simulink model "segway_planar_sim"  (R2023a)
settings: Solver=VariableStepAuto  StartTime=0.0  StopTime=5.0  RelTol=1e-3
values from neighbouring files (symbols this model uses):
  Cr2w = Cw2r^-1    [segway_ini.m]    (also in segway_planar_ini.m)
  Cw2r = [p.r/2     p.r/2;          p.r/p.b, -p.r/p.b]    [segway_ini.m]    (also in segway_planar_ini.m = [p.r])
  Ki = K(:,5:6)    [segway_ini.m]    (also in segway_planar_ini.m = K(:,4))
  Kx = K(:,1:4)    [segway_ini.m]    (also in segway_planar_ini.m = K(:,1:3))
  p = get_segway_params()    [segway_ini.m]    (also in segway_planar_ini.m)
  s = 2*pi    (= 6.28318530718)    [segway_planar_ini.m]
libraries: cstblocks x2
settings Model: Creator=Michael Peter  LastModifiedBy=Michael Peter

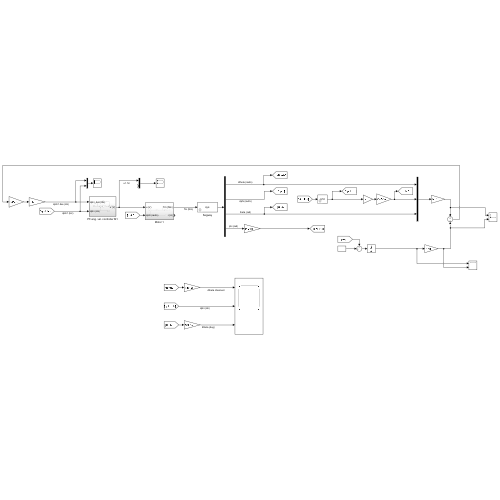
[thumbnail: Simulink's stored preview of the top-level diagram]
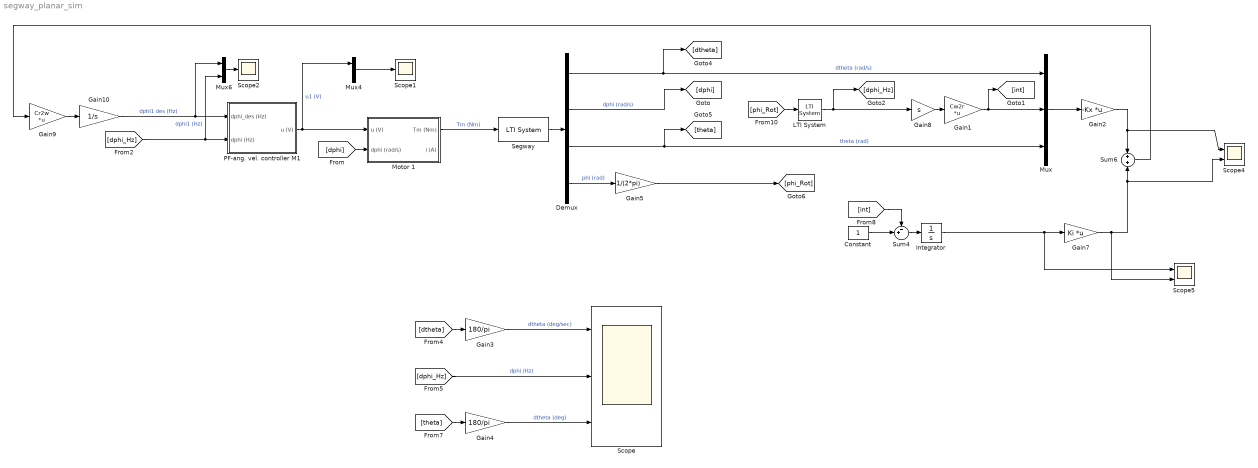
== system segway_planar_sim ==
  Constant : Constant
  Demux : Demux
  Gain1 : Gain  Gain=Cw2r  Multiplication=Matrix(K*u)
  Gain10 : Gain  Gain=1/s
  Gain2 : Gain  Gain=-Kx  Multiplication=Matrix(K*u)
  Gain3 : Gain  Gain=180/pi
  Gain4 : Gain  Gain=180/pi
  Gain5 : Gain  Gain=1/(2*pi)
  Gain7 : Gain  Gain=Ki  Multiplication=Matrix(K*u)
  Gain8 : Gain  Gain=s
  Gain9 : Gain  Gain=Cr2w  Multiplication=Matrix(K*u)
  Integrator : Integrator
  LTI System : cstblocks/LTI System  sys=Gfd  IC=[]
  Motor 1 : Subsystem
  Mux : Mux  Inputs=3
  Mux4 : Mux  Inputs=2
  Mux6 : Mux  Inputs=2
  PF-ang. vel. controller M1 : Subsystem
  Scope : Scope  NumInputPorts=3
  Scope1 : Scope
  Scope2 : Scope
  Scope4 : Scope  NumInputPorts=2
  Scope5 : Scope  NumInputPorts=2
  Segway : cstblocks/LTI System  sys=sys  IC=x0
  Sum4 : Sum  Inputs=-+|
  Sum6 : Sum  Inputs=+|+
  wires:
  Mux/1 -> Gain2/1
  Demux/2 -> [dphi]  "dphi (rad/s)"
  Segway/1 -> Demux/1
  Demux/3 -> [theta], Mux/3  "theta (rad)"
  Demux/1 -> [dtheta], Mux/1  "dtheta (rad/s)"
  Demux/4 -> Gain5/1  "phi (rad)"
  Sum4/1 -> Integrator/1
  Integrator/1 -> Scope5/1, Gain7/1
  [dtheta] -> Gain3/1
  [dphi_Hz] -> Scope/2  "dphi (Hz)"
  [theta] -> Gain4/1
  Gain3/1 -> Scope/1  "dtheta (deg/sec)"
  Gain4/1 -> Scope/3  "dtheta (deg)"
  Gain7/1 -> Scope5/2, Scope4/2, Sum6/2
  [int] -> Sum4/1
  [phi_Rot] -> LTI System/1
  Gain2/1 -> Sum6/1, Scope4/1
  LTI System/1 -> Gain8/1, [dphi_Hz]
  Constant/1 -> Sum4/2
  Sum6/1 -> Gain9/1
  Mux6/1 -> Scope2/1
  Motor 1/1(Tm (Nm)) -> Segway/1  "Tm (Nm)"
  PF-ang. vel. controller M1/1(u (V)) -> Mux4/1, Motor 1/1(u (V))  "u1 (V)"
  [dphi_Hz] -> PF-ang. vel. controller M1/2(dphi (Hz)), Mux6/2  "dphi1 (Hz)"
  Gain10/1 -> PF-ang. vel. controller M1/1(dphi_des (Hz)), Mux6/1  "dphi1 des (Hz)"
  [dphi] -> Motor 1/2(dphi (rad/s))
  Mux4/1 -> Scope1/1
  Gain8/1 -> Gain1/1
  Gain1/1 -> [int], Mux/2
  Gain5/1 -> [phi_Rot]
  Gain9/1 -> Gain10/1

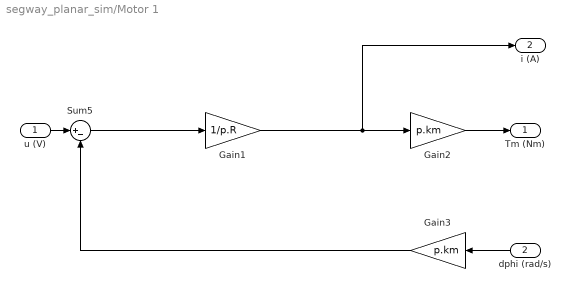
== system segway_planar_sim/Motor 1 ==
  u (V) : Inport
  dphi (rad/s) : Inport  Port=2
  Gain1 : Gain  Gain=1/p.R
  Gain2 : Gain  Gain=p.km
  Gain3 : Gain  Gain=p.km
  Sum5 : Sum  Inputs=|+-
  Tm (Nm) : Outport
  i (A) : Outport  Port=2
  wires:
  Gain1/1 -> i (A)/1, Gain2/1
  Gain3/1 -> Sum5/2
  u (V)/1 -> Sum5/1
  Sum5/1 -> Gain1/1
  dphi (rad/s)/1 -> Gain3/1
  Gain2/1 -> Tm (Nm)/1

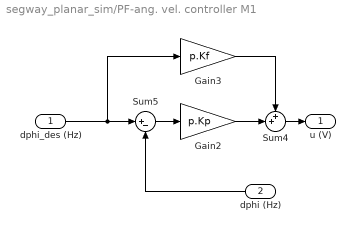
== system segway_planar_sim/PF-ang. vel. controller M1 ==
  dphi_des (Hz) : Inport
  dphi (Hz) : Inport  Port=2
  Gain2 : Gain  Gain=p.Kp
  Gain3 : Gain  Gain=p.Kf
  Sum4 : Sum  Inputs=++|
  Sum5 : Sum  Inputs=|+-
  u (V) : Outport
  wires:
  Sum5/1 -> Gain2/1
  dphi_des (Hz)/1 -> Gain3/1, Sum5/1
  dphi (Hz)/1 -> Sum5/2
  Gain3/1 -> Sum4/1
  Gain2/1 -> Sum4/2
  Sum4/1 -> u (V)/1
